simulink model "test_attention"  (Simulink 8.0)
settings: Solver=FixedStepDiscrete  StartTime=0.0  StopTime=Inf  FixedStep=.001  RelTol=1e-3
libraries: simulink x4
CloseFcn:
  | rtwprivate ssgencode ModelCloseRequest rwalk_multi_local_v1
settings Model: Creator=limblab  LastModifiedBy=ricardo  ParamWorkspaceSource=ReferencedWorkspace  ExtModeArmWhenConnect=off  BufferReuse=off
settings DataIOCC: LimitDataPoints=off  SaveFormat=StructureWithTime  SignalLoggingSaveFormat=ModelDataLogs  SaveState=on  SignalLoggingName=sigsOut
settings OptimizationCC: BlockReduction=off  BooleanDataType=off  OptimizeBlockIOStorage=off  BufferReuse=off  ExpressionFolding=off  FoldNonRolledExpr=off  LocalBlockOutputs=off  InitFltsAndDblsToZero=on
settings DebuggingCC: SaveWithParameterizedLinksMsg=none  SignalResolutionControl=TryResolveAllWithWarning  SolverPrmCheckMsg=none  MultiTaskDSMMsg=warning  MultiTaskCondExecSysMsg=none  FcnCallInpInsideContextMsg=UseLocalSettings  StrictBusMsg=None
settings HardwareCC: ProdIntDivRoundTo=Zero  ProdEndianess=LittleEndian  ProdHWDeviceType=Generic->32-bit x86 compatible  TargetIntDivRoundTo=Zero  TargetEndianess=LittleEndian  TargetHWDeviceType=32-bit xPC Target (Intel Pentium)
settings SFSimCC: SimParseCustomCode=off
settings RTWCC: SystemTargetFile=xpctarget.tlc  TemplateMakefile=xpc_default_tmf  Description=xPC Target  GenerateReport=on  ProcessScript=xpctarget_make_rtw_hook  IncludeERTFirstTime=on
settings xpcTargetCC: TargetFcnLib=ansi_tfl_tmw.mat  CodeReplacementLibrary=XPC_BLAS  ParMdlRefBuildCompliant=on  ConcurrentExecutionCompliant=on  CombineSignalStateStructs=off  GRTInterface=on  xPCTaskExecutionProfile=off  xPCRL32EventNumber=5000  xPCisDownloadable=off  xPCLoadParamSetFile=off  xPCConcurrentTasks=off  xPCEnableSFAnimation=off

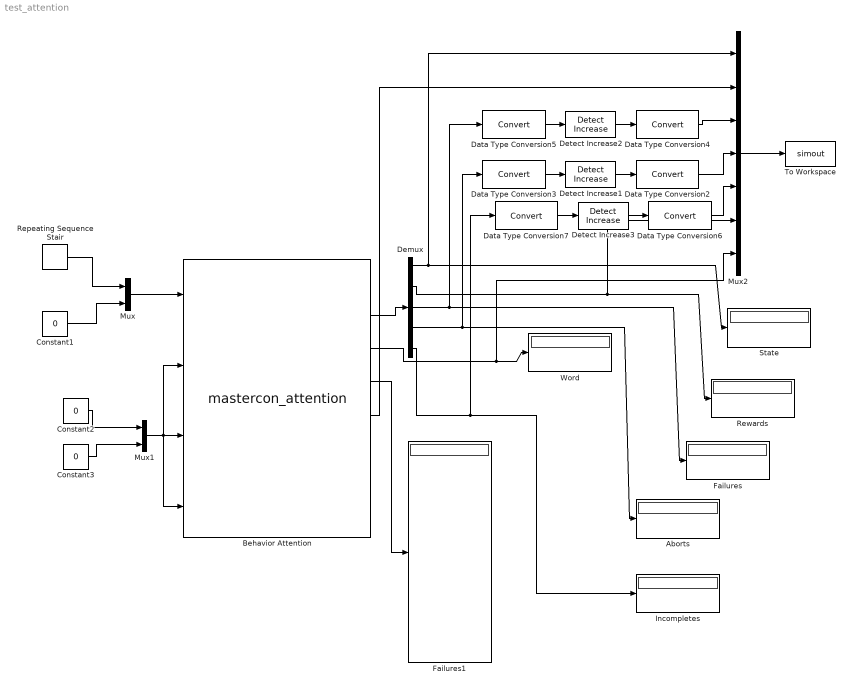
== system test_attention ==
  Aborts : Display
  Behavior Attention : S-Function  FunctionName=mastercon_attention  Parameters="0 .5 1 5 1 1 1   3 10   50 50 10 0 0 1 1 4 0   1 10 80 1 50 .1 0 1.57 3.14 5 0 1.57   .3 5 1.57 3.14 0 1.57 .005   1 1 .003 0 .2 0 0"  EnableBusSupport=off
      mask Display:
      | disp('Master Control')
      | port_label('input',1,'pos')
      | port_label('input',2,'offsets')
      | port_label('input',3,'force')
      | port_label('input',4,'catch force')
      | port_label('output',1,'force')
      | port_label('output',2,'status')
      | port_label('output',3,'word')
      | port_label('output',4,'targets')
      | port_label('output',5,'reward')
      | port_label('output',6,'tone')
      | port_label('output',7,'version')
      | port_label('output',8,'pos')
  Constant1 : Constant  Value=0
  Constant2 : Constant  Value=0
  Constant3 : Constant  Value=0
  Data Type Conversion{2..7} (6 alike) : DataTypeConversion
  Demux : Demux  Outputs=5
  Detect Increase1 : simulink/Logic and Bit Operations/Detect Increase  vinit=0.0  InputProcessing=Inherited  OutDataTypeStr=uint8
  Detect Increase2 : simulink/Logic and Bit Operations/Detect Increase  vinit=0.0  InputProcessing=Inherited  OutDataTypeStr=uint8
  Detect Increase3 : simulink/Logic and Bit Operations/Detect Increase  vinit=0.0  InputProcessing=Inherited  OutDataTypeStr=uint8
  Failures : Display
  Failures1 : Display
  Incompletes : Display
  Mux : Mux  Inputs=2
  Mux1 : Mux  Inputs=2
  Mux2 : Mux  Inputs=7
  Repeating Sequence Stair : simulink/Sources/Repeating Sequence Stair  OutValues=[0 -10 0 0 10 0].'  tsamp=1  OutMin=[]  OutMax=[]  OutDataTypeStr=float('double')  OutputDataTypeScalingMode=Specify via dialog  OutDataType=float('double')  ConRadixGroup=Best Precision: Vector-wise  OutScaling=2^-12
  Rewards : Display
  State : Display
  To Workspace : ToWorkspace  VariableName=simout  SampleTime=-1  SaveFormat=Structure
  Word : Display
  wires:
  Constant1/1 -> Mux/2
  Mux/1 -> Behavior Attention/1
  Behavior Attention/2 -> Demux/1
  Demux/1 -> State/1, Mux2/1
  Constant2/1 -> Mux1/1
  Constant3/1 -> Mux1/2
  Mux1/1 -> Behavior Attention/4, Behavior Attention/2, Behavior Attention/3
  Demux/2 -> Rewards/1, Mux2/6
  Demux/3 -> Failures/1, Data Type Conversion5/1
  Behavior Attention/4 -> Failures1/1
  Demux/5 -> Incompletes/1, Data Type Conversion7/1
  Demux/4 -> Aborts/1, Data Type Conversion3/1
  Mux2/1 -> To Workspace/1
  Data Type Conversion3/1 -> Detect Increase1/1
  Detect Increase1/1 -> Data Type Conversion2/1
  Data Type Conversion5/1 -> Detect Increase2/1
  Detect Increase2/1 -> Data Type Conversion4/1
  Data Type Conversion4/1 -> Mux2/3
  Data Type Conversion2/1 -> Mux2/4
  Data Type Conversion7/1 -> Detect Increase3/1
  Detect Increase3/1 -> Data Type Conversion6/1
  Data Type Conversion6/1 -> Mux2/5
  Behavior Attention/5 -> Mux2/2
  Repeating Sequence Stair/1 -> Mux/1
  Behavior Attention/3 -> Mux2/7, Word/1
